simulink model "CuttingSim"  (R2021a)
settings: Solver=FixedStepAuto  StartTime=0.0  StopTime=Inf  RelTol=1e-3  EnableMultiTasking=on
model workspace (MAT data in the model file):
  SL_ROS_VariableLengthArrays_MaxSizes.CommonInfo.ArrayTruncateAction = 'EmitWarning'
  SL_ROS_VariableLengthArrays_MaxSizes.MsgTypeMap = containers.Map
  SL_ROS_VariableLengthArrays_MaxSizes.MsgTypeMap.serialization.keys = {'std_msgs/Float64MultiArray'}
  SL_ROS_VariableLengthArrays_MaxSizes.MsgTypeMap.serialization.values{1}.PropertyName = 'Data'
  SL_ROS_VariableLengthArrays_MaxSizes.MsgTypeMap.serialization.values{1}.DataType = 'double'
  SL_ROS_VariableLengthArrays_MaxSizes.MsgTypeMap.serialization.values{1}.MaxLength = 7
  SL_ROS_VariableLengthArrays_MaxSizes.MsgTypeMap.serialization.uniformity = 0
  SL_ROS_VariableLengthArrays_MaxSizes.MsgTypeMap.serialization.keyType = 'char'
  SL_ROS_VariableLengthArrays_MaxSizes.MsgTypeMap.serialization.valueType = 'any'
  q0 = Simulink.Parameter
  q0.Value = [-0.8706; 0.1348; 0.656; -1.7221; -0.0873; 1.3219; -0.1965]
  q0.DataType = 'auto'
  q0.Dimensions = [7 1]
  v_limit = 0.05
values from neighbouring files (symbols this model uses):
  Tf = 10    [createAgent.m]
  Ts = 0.02    [createAgent.m]
undefined symbols (not defined in the file or in its folder): rl
libraries: simulink x26, robotlib x8, vrlib x1, dspinverses x1, rllib x1, dspmathops x1
settings Model: ExtModeTrigMode=oneshot  ExtModeArmWhenConnect=off  Creator=pic  LastModifiedBy=workcell
settings SolverCC: AlgebraicLoopSolver=TrustRegion
settings DataIOCC: SaveFormat=StructureWithTime  SignalLoggingSaveFormat=ModelDataLogs
settings OptimizationCC: BlockReduction=off  BooleanDataType=off  EnhancedBackFolding=on  PassReuseOutputArgsThreshold=0  ExpressionDepthLimit=2147483647  InitFltsAndDblsToZero=on  MaxStackSize=64  OptimizeBlockOrder=speed  DifferentSizesBufferReuse=on  OptimizationCustomize=off
settings DebuggingCC: SaveWithParameterizedLinksMsg=none  UnderspecifiedInitializationDetection=Classic  MergeDetectMultiDrivingBlocksExec=none  SignalResolutionControl=TryResolveAllWithWarning  MultiTaskDSMMsg=warning  MultiTaskCondExecSysMsg=none  ParameterTunabilityLossMsg=error  FcnCallInpInsideContextMsg=warning  AllowSymbolicDim=off  StateNameClashWarn=warning  SFUnexpectedBacktrackingDiag=warning  SFNoUnconditionalDefaultTransitionDiag=warning  SFExecutionAtInitializationDiag=none  SFMachineParentedDataDiag=warning  ArithmeticOperatorsInVariantConditions=warning
settings HardwareCC: ProdBitPerPointer=32  ProdBitPerSizeT=32  ProdBitPerPtrDiffT=32  ProdLargestAtomicFloat=None  ProdIntDivRoundTo=Undefined  ProdEndianess=Unspecified  ProdWordSize=32  ProdHWDeviceType=Generic->Unspecified (assume 32-bit Generic)  TargetUnknown=on  UseEmbeddedCoderFeatures=off
settings ModelReferenceCC: PropagateSignalLabelsOutOfModel=off
settings SFSimCC: SimUseLocalCustomCode=off  MATLABDynamicMemAlloc=off  CustomCodeUndefinedFunction=UseInterfaceOnly  SimTargetLang=C++
settings RTWCC: SystemTargetFile=ert.tlc  HardwareBoard=Robot Operating System (ROS)  TLCOptions="-aInlineSetEventsForThisBaseRateFcn=TLC_FALSE -aSuppressMultiTaskScheduler=TLC_FALSE  -aRateBasedStepFcn=0"  TemplateMakefile=ert_default_tmf  RTWUseLocalCustomCode=off  Toolchain=Catkin  TargetLang=C++
settings CodeAppCC: ForceParamTrailComments=on  OperatorAnnotations=on
settings ERTTargetCC: ERTCustomFileBanners=off  SupportContinuousTime=on  SupportNonInlinedSFcns=on  RemoveResetFunc=off  ModelStepFunctionPrototypeControlCompliant=off
settings ConfigComp: CovMetricSettings=dw  CovSaveCumulativeToWorkspaceVar=on  CovSaveSingleToWorkspaceVar=on  CovExternalEMLEnable=off  CovSFcnEnable=off

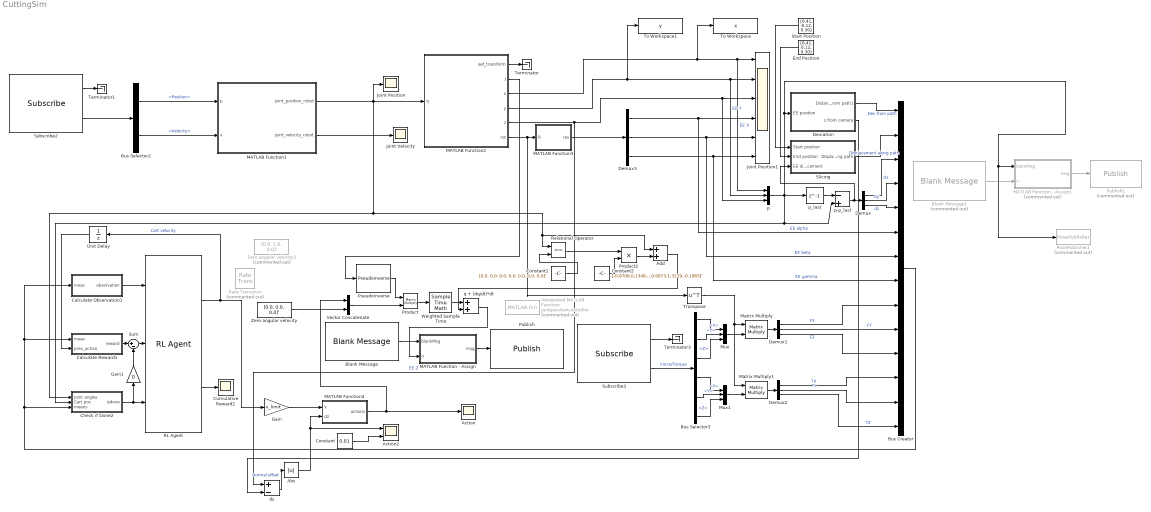
== system CuttingSim ==
  Abs : Abs
  Action : Scope
  Action2 : Scope  NumInputPorts=2
  Add : Sum
  Blank Message : robotlib/Blank Message  messageClass=Message  entityType=std_msgs/Float64MultiArray  messageType=std_msgs/Float64MultiArray  SampleTime=inf  legacyBusStruct=off
  Blank Message1 : robotlib/Blank Message  Commented=on  messageClass=Message  entityType=geometry_msgs/PoseStamped  messageType=geometry_msgs/PoseStamped  SampleTime=inf  legacyBusStruct=off
  Bus Creator : BusCreator  Inputs=14
  Bus Selector2 : BusSelector  OutputSignals=Position,Velocity
  Bus Selector3 : BusSelector  OutputSignals=Wrench.Force.X,Wrench.Force.Y,Wrench.Force.Z,Wrench.Torque.X,Wrench.Torque.Y,Wrench.Torque.Z
  Calculate Observation1 : Subsystem
  Calculate Reward1 : Subsystem
  Check if Done2 : Subsystem
  Constant : Constant  Value=0.01
  Constant1 : Constant  Value=[0.0, 0.0, 0.0, 0.0, 0.0, 0.0, 0.0]'
  Constant2 : Constant  Value=[-0.8706,0.1348,0.6560,-1.7221,-0.0873,1.3219,-0.1965]'
  Cumulative Reward2 : Scope
  Demux{,1..3} (4 alike) : Demux  Outputs=3
  Deviation : Subsystem
  End Position : Constant  Value=[0.41, 0.12, 0.30]  VectorParams1D=off
  Gain : Gain  Gain=v_limit
  Gain1 : Gain  Gain=0
  Interpreted MATLAB Function : MATLABFcn  Commented=on  MATLABFcn=jointpositioncontroller  OutputDimensions=0
  Joint Position : Scope
  Joint Position1 : Scope  NumInputPorts=6
  Joint Velocity : Scope
  MATLAB Function - Assign : MATLAB Function  TreatAsAtomicUnit=on
  MATLAB Function - Assign1 : MATLAB Function  Commented=on  TreatAsAtomicUnit=on
  MATLAB Function1 : MATLAB Function  TreatAsAtomicUnit=on
  MATLAB Function2 : MATLAB Function  TreatAsAtomicUnit=on
  MATLAB Function3 : MATLAB Function  TreatAsAtomicUnit=on
  MATLAB Function4 : MATLAB Function  TreatAsAtomicUnit=on
  Matrix Multiply : Product  Multiplication=Matrix(*)
  Matrix Multiply1 : Product  Multiplication=Matrix(*)
  Mux : Mux  Inputs=3
  Mux1 : Mux  Inputs=3
  PosePublisher1 : MATLABFcn  Commented=on  MATLABFcn=PosePublisher  OutputDimensions=0
  Product : Product  Multiplication=Matrix(*)
  Product2 : Product
  Pseudoinverse : dspinverses/Pseudoinverse  wanterr=off  SimulateUsing=Interpreted execution
      settings: SourceProductBaseCode=DS
  Publish : robotlib/Publish  topicSource=Select from ROS network  topic=/iiwa/PositionJointInterface_group_controller/command  messageType=std_msgs/Float64MultiArray  legacyBusStruct=off  messageQueueLength=1
  Publish1 : robotlib/Publish  Commented=on  topicSource=Select from ROS network  topic=/iiwa/PositionJointInterface_cutting_controller/CartesianPose  messageType=geometry_msgs/PoseStamped  legacyBusStruct=off  messageQueueLength=1
  RL Agent : rllib/RL Agent  Agent=rl.util.PolicyInstance.get('CuttingSim/RL Agent')  ExternalActionAsInput=off  ProvideCumRwd=on  TreatAsDirectFeedthrough=on
      settings: SourceProductName=Reinforcement Learning
  Rate Transition : RateTransition  Commented=on
  Relational Operator : RelationalOperator  Operator===  OutDataTypeStr=boolean  RndMeth=Simplest
  Slicing : Subsystem
  Start Position : Constant  Value=[0.41, -0.12, 0.30]  VectorParams1D=off
  Subscribe2 : robotlib/Subscribe  topicSource=Select from ROS network  topic=/iiwa/joint_states  messageType=sensor_msgs/JointState  SampleTime=-1  legacyBusStruct=off  messageQueueLength=1
  Subscribe3 : robotlib/Subscribe  topicSource=Select from ROS network  topic=/iiwa/CartesianWrench  messageType=geometry_msgs/WrenchStamped  SampleTime=-1  legacyBusStruct=off  messageQueueLength=1
  Sum : Sum  Inputs=|+-
  Terminator : Terminator
  Terminator1 : Terminator
  Terminator3 : Terminator
  To Workspace : ToWorkspace  VariableName=x  SaveFormat=Timeseries  SampleTime=-1
  To Workspace1 : ToWorkspace  VariableName=y  SaveFormat=Timeseries  SampleTime=-1
  Transpose : Math  Operator=transpose  SaturateOnIntegerOverflow=on
  Unit Delay : UnitDelay  SampleTime=-1  HasFrameUpgradeWarning=on
  Vector Concatenate : Concatenate
  Weighted Sample Time : SampleTimeMath  TsampMathOp=*
  Zero angular velocity : Constant  Value=[0.0, 0.0, 0.0]'
  Zero angular velocity1 : Constant  Commented=on  Value=[0.0, 1.0, 0.0]'
  dz : Sum  Inputs=+-
  p : Mux  Inputs=3
  p-p_last : Sum  Inputs=-+
  p_last : Delay  DelayLength=1  InitialCondition=0
  q + (dq/dt)*dt : Sum
  wires:
  Bus Creator/1 -> Check if Done2/3(means), Calculate Observation1/1(meas), Calculate Reward1/1(meas)
  Calculate Observation1/1(observation) -> RL Agent/1
  Check if Done2/1(isdone) -> RL Agent/3, Gain1/1
  RL Agent/1 -> Gain/1, Unit Delay/1  "Cart velocity"
  RL Agent/2 -> Cumulative Reward2/1
  Subscribe3/1 -> Terminator3/1
  Subscribe3/2 -> Bus Selector3/1  "Force/Torque"
  MATLAB Function2/3(x) -> To Workspace/1, Joint Position1/1, p/1  "EE X"
  MATLAB Function2/4(y) -> Joint Position1/2, p/2, To Workspace1/1  "EE Y"
  MATLAB Function2/5(z) -> p/3, Joint Position1/3, dz/1  "EE Z"
  Demux3/1 -> Bus Creator/6, Joint Position1/4  "EE alpha"
  Demux3/2 -> Bus Creator/7, Joint Position1/5  "EE beta"
  Demux3/3 -> Bus Creator/8, Joint Position1/6  "EE gamma"
  MATLAB Function2/6(rot) -> Transpose/1, MATLAB Function3/1(R)
  MATLAB Function3/1(res) -> Demux3/1
  Product/1 -> Weighted Sample Time/1
  Pseudoinverse/1 -> Product/1
  MATLAB Function2/2(J) -> Pseudoinverse/1
  Unit Delay/1 -> Calculate Reward1/2(prev_action)
  MATLAB Function2/1(eef_transform) -> Terminator/1
  p/1 -> PosePublisher1/1, MATLAB Function - Assign1/1(blankMsg), Deviation/1(EE position), Check if Done2/2(Cart pos), p-p_last/2, p_last/1
  End Position/1 -> Slicing/2(End position)
  Start Position/1 -> Slicing/1(Start position)
  Slicing/1(Displacement along path) -> Bus Creator/2  "Displacement along path"
  Deviation/1(Distance from path1) -> Bus Creator/1  "Dev from path"
  p_last/1 -> p-p_last/1
  p-p_last/1 -> Slicing/3(EE displacement), Demux/1
  Demux/1 -> Bus Creator/3  "dx"
  Demux/2 -> Bus Creator/4  "dy"
  Demux/3 -> Bus Creator/5  "dz"
  MATLAB Function1/1(joint_position_robot) -> Relational Operator/1, Add/1, Check if Done2/1(Joint angles), MATLAB Function2/1(q), Joint Position/1
  Subscribe2/2 -> Bus Selector2/1
  Bus Selector2/2 -> MATLAB Function1/2(v)  "<Velocity>"
  Bus Selector2/1 -> MATLAB Function1/1(p)  "<Position>"
  MATLAB Function1/2(joint_velocity_robot) -> Joint Velocity/1
  MATLAB Function - Assign/1(msg) -> Publish/1
  Blank Message/1 -> MATLAB Function - Assign/1(blankMsg)
  Subscribe2/1 -> Terminator1/1
  Bus Selector3/4 -> Mux1/1  "<X>"
  Bus Selector3/5 -> Mux1/2  "<Y>"
  Bus Selector3/6 -> Mux1/3  "<Z>"
  Bus Selector3/1 -> Mux/1  "<X>"
  Bus Selector3/2 -> Mux/2  "<Y>"
  Bus Selector3/3 -> Mux/3  "<Z>"
  Mux1/1 -> Matrix Multiply1/2
  Mux/1 -> Matrix Multiply/2
  Matrix Multiply1/1 -> Demux2/1
  Matrix Multiply/1 -> Demux1/1
  Demux1/1 -> Bus Creator/9  "FX"
  Demux1/2 -> Bus Creator/10  "FY"
  Demux1/3 -> Bus Creator/11  "FZ"
  Demux2/1 -> Bus Creator/12  "TX"
  Demux2/3 -> Bus Creator/14  "TZ"
  Demux2/2 -> Bus Creator/13  "TY"
  Transpose/1 -> Matrix Multiply1/1, Matrix Multiply/1
  Constant1/1 -> Relational Operator/2
  Relational Operator/1 -> Product2/1
  Product2/1 -> Add/2
  Constant2/1 -> Product2/2
  Add/1 -> q + (dq/dt)*dt/2
  Calculate Reward1/1(reward) -> Sum/1
  Sum/1 -> RL Agent/2
  Gain1/1 -> Sum/2
  Zero angular velocity/1 -> Vector Concatenate/2
  Vector Concatenate/1 -> Product/2
  Weighted Sample Time/1 -> q + (dq/dt)*dt/1
  q + (dq/dt)*dt/1 -> MATLAB Function - Assign/2(u)
  MATLAB Function - Assign1/1(msg) -> Publish1/1
  Blank Message1/1 -> MATLAB Function - Assign1/2(u)
  Deviation/2(z from camera) -> dz/2
  MATLAB Function4/1(actions) -> Vector Concatenate/1, Action/1
  Gain/1 -> MATLAB Function4/1(v)
  Abs/1 -> Action2/1, MATLAB Function4/2(dz)
  dz/1 -> Abs/1  "Normal offset"
  Constant/1 -> Action2/2

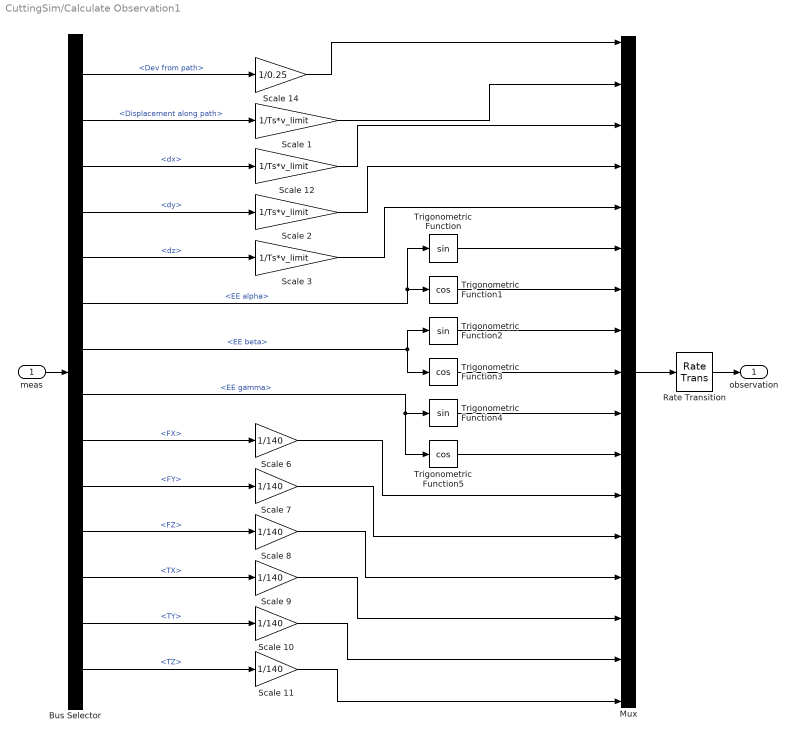
== system CuttingSim/Calculate Observation1 ==
  meas : Inport
  Bus Selector : BusSelector  OutputSignals=Dev from path,Displacement along path,dx,dy,dz,EE alpha,EE beta,EE gamma,FX,FY,FZ,TX,TY,TZ
  Mux : Mux  Inputs=17
  Rate Transition : RateTransition
  Scale {1..3,12} (4 alike) : Gain  Gain=1/Ts*v_limit
  Scale {6..11} (6 alike) : Gain  Gain=1/140
  Scale 14 : Gain  Gain=1/0.25
  Trigonometric Function : Trigonometry
  Trigonometric Function1 : Trigonometry  Operator=cos
  Trigonometric Function2 : Trigonometry
  Trigonometric Function3 : Trigonometry  Operator=cos
  Trigonometric Function4 : Trigonometry
  Trigonometric Function5 : Trigonometry  Operator=cos
  observation : Outport  VectorParamsAs1DForOutWhenUnconnected=off
  wires:
  meas/1 -> Bus Selector/1
  Mux/1 -> Rate Transition/1
  Bus Selector/1 -> Scale 14/1  "<Dev from path>"
  Scale 14/1 -> Mux/1
  Bus Selector/2 -> Scale 1/1  "<Displacement along path>"
  Scale 1/1 -> Mux/2
  Bus Selector/6 -> Trigonometric Function/1, Trigonometric Function1/1  "<EE alpha>"
  Bus Selector/7 -> Trigonometric Function2/1, Trigonometric Function3/1  "<EE beta>"
  Bus Selector/8 -> Trigonometric Function5/1, Trigonometric Function4/1  "<EE gamma>"
  Bus Selector/9 -> Scale 6/1  "<FX>"
  Trigonometric Function/1 -> Mux/6
  Trigonometric Function1/1 -> Mux/7
  Trigonometric Function2/1 -> Mux/8
  Trigonometric Function3/1 -> Mux/9
  Trigonometric Function5/1 -> Mux/11
  Trigonometric Function4/1 -> Mux/10
  Scale 6/1 -> Mux/12
  Rate Transition/1 -> observation/1
  Bus Selector/10 -> Scale 7/1  "<FY>"
  Scale 7/1 -> Mux/13
  Bus Selector/11 -> Scale 8/1  "<FZ>"
  Bus Selector/12 -> Scale 9/1  "<TX>"
  Bus Selector/13 -> Scale 10/1  "<TY>"
  Bus Selector/14 -> Scale 11/1  "<TZ>"
  Scale 8/1 -> Mux/14
  Scale 9/1 -> Mux/15
  Scale 10/1 -> Mux/16
  Scale 11/1 -> Mux/17
  Scale 12/1 -> Mux/3
  Bus Selector/3 -> Scale 12/1  "<dx>"
  Bus Selector/4 -> Scale 2/1  "<dy>"
  Bus Selector/5 -> Scale 3/1  "<dz>"
  Scale 2/1 -> Mux/4
  Scale 3/1 -> Mux/5

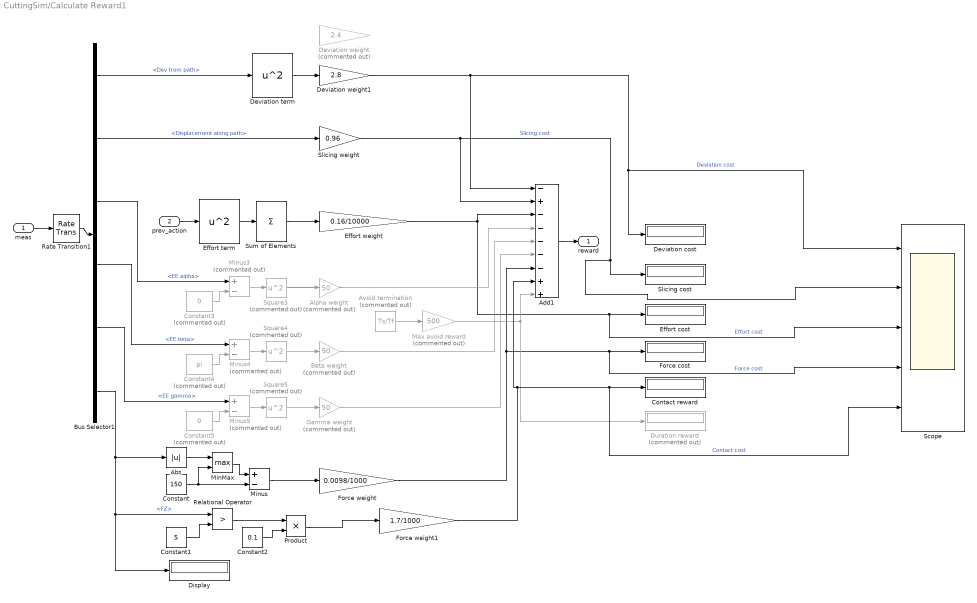
== system CuttingSim/Calculate Reward1 ==
  meas : Inport
  prev_action : Inport  Port=2
  Abs : Abs
  Add1 : Sum  Inputs=-+-----++
  Alpha weight : Gain  Commented=on  Gain=50
  Avoid termination : Constant  Commented=on  Value=Ts/Tf
  Beta weight : Gain  Commented=on  Gain=50
  Bus Selector1 : BusSelector  OutputSignals=Dev from path,Displacement along path,EE alpha,EE beta,EE gamma,FZ
  Constant : Constant  Value=150
  Constant1 : Constant  Value=5
  Constant2 : Constant  Value=0.1
  Constant3 : Constant  Commented=on  Value=0
  Constant4 : Constant  Commented=on  Value=pi
  Constant5 : Constant  Commented=on  Value=0
  Contact reward : Display
  Deviation cost : Display
  Deviation term : Math  Operator=square  SaturateOnIntegerOverflow=on
  Deviation weight : Gain  Commented=on  Gain=2.4
  Deviation weight1 : Gain  Gain=2.8
  Display : Display
  Duration reward : Display  Commented=on
  Effort cost : Display
  Effort term : Math  Operator=square  SaturateOnIntegerOverflow=on
  Effort weight : Gain  Gain=0.16/10000
  Force cost : Display
  Force weight : Gain  Gain=0.0098/1000
  Force weight1 : Gain  Gain=1.7/1000
  Gamma weight : Gain  Commented=on  Gain=50
  Max avoid reward : Gain  Commented=on  Gain=500
  MinMax : MinMax  Function=max  Inputs=2
  Minus : Sum  Inputs=+-
  Minus3 : Sum  Commented=on  Inputs=+-
  Minus4 : Sum  Commented=on  Inputs=+-
  Minus5 : Sum  Commented=on  Inputs=+-
  Product : Product
  Rate Transition1 : RateTransition  OutPortSampleTime=Ts
  Relational Operator : RelationalOperator  Operator=>  OutDataTypeStr=boolean  RndMeth=Simplest
  Scope : Scope  NumInputPorts=5
  Slicing cost : Display
  Slicing weight : Gain  Gain=0.96
  Square3 : Math  Commented=on  Operator=square  SignedPower=on  SaturateOnIntegerOverflow=on
  Square4 : Math  Commented=on  Operator=square  SignedPower=on  SaturateOnIntegerOverflow=on
  Square5 : Math  Commented=on  Operator=square  SignedPower=on  SaturateOnIntegerOverflow=on
  Sum of Elements : Sum  Inputs=+
  reward : Outport  VectorParamsAs1DForOutWhenUnconnected=off
  wires:
  meas/1 -> Rate Transition1/1
  Rate Transition1/1 -> Bus Selector1/1
  Add1/1 -> reward/1
  Minus3/1 -> Square3/1
  Constant3/1 -> Minus3/2
  Bus Selector1/3 -> Minus3/1  "<EE alpha>"
  Bus Selector1/4 -> Minus4/1  "<EE beta>"
  Constant4/1 -> Minus4/2
  Minus4/1 -> Square4/1
  Minus5/1 -> Square5/1
  Constant5/1 -> Minus5/2
  Bus Selector1/5 -> Minus5/1  "<EE gamma>"
  Sum of Elements/1 -> Effort weight/1
  Square3/1 -> Alpha weight/1
  Square4/1 -> Beta weight/1
  Square5/1 -> Gamma weight/1
  prev_action/1 -> Effort term/1
  Effort weight/1 -> Scope/3, Effort cost/1, Add1/3  "Effort cost"
  Deviation weight1/1 -> Add1/1, Scope/1, Deviation cost/1  "Deviation cost"
  Deviation term/1 -> Deviation weight1/1
  Bus Selector1/2 -> Slicing weight/1  "<Displacement along path>"
  Bus Selector1/1 -> Deviation term/1  "<Dev from path>"
  Effort term/1 -> Sum of Elements/1
  Bus Selector1/6 -> Relational Operator/1, Display/1, Abs/1  "<FZ>"
  Constant/1 -> Minus/2, MinMax/2
  Abs/1 -> MinMax/1
  MinMax/1 -> Minus/1
  Minus/1 -> Force weight/1
  Force weight/1 -> Add1/7, Scope/4, Force cost/1  "Force cost"
  Constant1/1 -> Relational Operator/2
  Relational Operator/1 -> Product/1
  Constant2/1 -> Product/2
  Product/1 -> Force weight1/1
  Alpha weight/1 -> Add1/4
  Beta weight/1 -> Add1/5
  Gamma weight/1 -> Add1/6
  Avoid termination/1 -> Max avoid reward/1
  Max avoid reward/1 -> Duration reward/1, Add1/9
  Force weight1/1 -> Add1/8, Scope/5, Contact reward/1  "Contact cost"
  Slicing weight/1 -> Add1/2, Scope/2, Slicing cost/1  "Slicing cost"

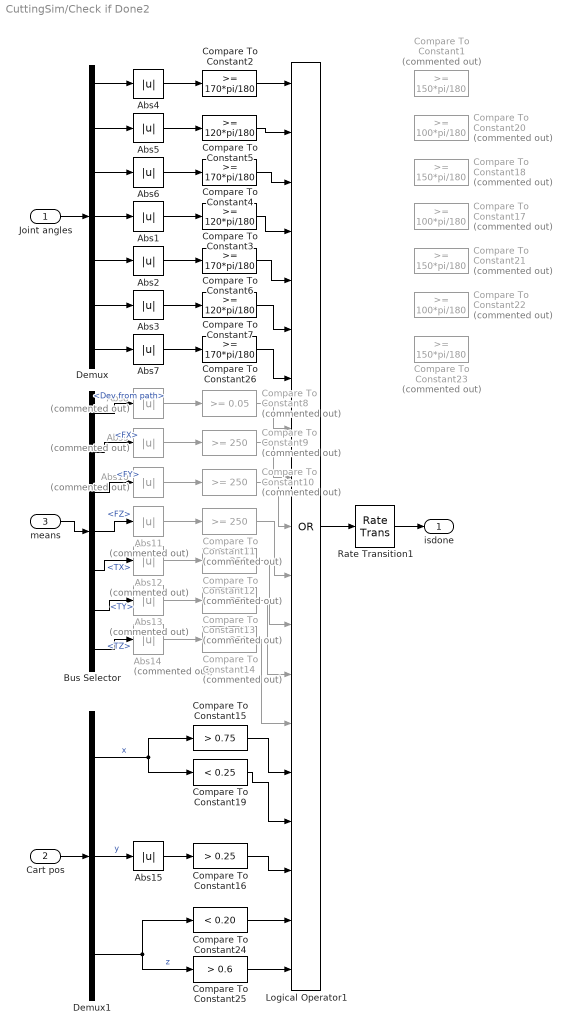
== system CuttingSim/Check if Done2 ==
  Joint angles : Inport
  Cart pos : Inport  Port=2
  means : Inport  Port=3
  Abs{1..7,15} (8 alike) : Abs
  Abs{8..14} (7 alike) : Abs  Commented=on
  Bus Selector : BusSelector  OutputSignals=Dev from path,FX,FY,FZ,TX,TY,TZ
  Compare To Constant{1,18,21,23} (4 alike) : simulink/Logic and Bit Operations/Compare To Constant  Commented=on  relop=>=  const=150*pi/180  OutDataTypeStr=boolean
  Compare To Constant{9..14} (6 alike) : simulink/Logic and Bit Operations/Compare To Constant  Commented=on  relop=>=  const=250  OutDataTypeStr=boolean
  Compare To Constant15 : simulink/Logic and Bit Operations/Compare To Constant  relop=>  const=0.75  OutDataTypeStr=boolean
  Compare To Constant16 : simulink/Logic and Bit Operations/Compare To Constant  relop=>  const=0.25  OutDataTypeStr=boolean
  Compare To Constant17 : simulink/Logic and Bit Operations/Compare To Constant  Commented=on  relop=>=  const=100*pi/180  OutDataTypeStr=boolean
  Compare To Constant19 : simulink/Logic and Bit Operations/Compare To Constant  relop=<  const=0.25  OutDataTypeStr=boolean
  Compare To Constant{2,4,6,26} (4 alike) : simulink/Logic and Bit Operations/Compare To Constant  relop=>=  const=170*pi/180  OutDataTypeStr=boolean
  Compare To Constant20 : simulink/Logic and Bit Operations/Compare To Constant  Commented=on  relop=>=  const=100*pi/180  OutDataTypeStr=boolean
  Compare To Constant22 : simulink/Logic and Bit Operations/Compare To Constant  Commented=on  relop=>=  const=100*pi/180  OutDataTypeStr=boolean
  Compare To Constant24 : simulink/Logic and Bit Operations/Compare To Constant  relop=<  const=0.20  OutDataTypeStr=boolean
  Compare To Constant25 : simulink/Logic and Bit Operations/Compare To Constant  relop=>  const=0.6  OutDataTypeStr=boolean
  Compare To Constant3 : simulink/Logic and Bit Operations/Compare To Constant  relop=>=  const=120*pi/180  OutDataTypeStr=boolean
  Compare To Constant5 : simulink/Logic and Bit Operations/Compare To Constant  relop=>=  const=120*pi/180  OutDataTypeStr=boolean
  Compare To Constant7 : simulink/Logic and Bit Operations/Compare To Constant  relop=>=  const=120*pi/180  OutDataTypeStr=boolean
  Compare To Constant8 : simulink/Logic and Bit Operations/Compare To Constant  Commented=on  relop=>=  const=0.05  OutDataTypeStr=boolean
  Demux : Demux  Outputs=7
  Demux1 : Demux  Outputs=3
  Logical Operator1 : Logic  Operator=OR  Inputs=19  AllPortsSameDT=off  OutDataTypeStr=boolean
  Rate Transition1 : RateTransition
  isdone : Outport  VectorParamsAs1DForOutWhenUnconnected=off
  wires:
  Compare To Constant8/1 -> Logical Operator1/8
  Demux/7 -> Abs7/1
  Compare To Constant26/1 -> Logical Operator1/7
  Demux/3 -> Abs6/1
  Demux/2 -> Abs5/1
  Abs3/1 -> Compare To Constant7/1
  Abs7/1 -> Compare To Constant26/1
  Compare To Constant3/1 -> Logical Operator1/4
  means/1 -> Bus Selector/1
  Abs8/1 -> Compare To Constant8/1
  Abs4/1 -> Compare To Constant2/1
  Demux/1 -> Abs4/1
  Rate Transition1/1 -> isdone/1
  Compare To Constant7/1 -> Logical Operator1/6
  Compare To Constant2/1 -> Logical Operator1/1
  Demux/5 -> Abs2/1
  Demux/6 -> Abs3/1
  Abs6/1 -> Compare To Constant4/1
  Abs2/1 -> Compare To Constant6/1
  Logical Operator1/1 -> Rate Transition1/1
  Compare To Constant5/1 -> Logical Operator1/2
  Abs1/1 -> Compare To Constant3/1
  Abs5/1 -> Compare To Constant5/1
  Compare To Constant6/1 -> Logical Operator1/5
  Joint angles/1 -> Demux/1
  Bus Selector/2 -> Abs9/1  "<FX>"
  Bus Selector/3 -> Abs10/1  "<FY>"
  Bus Selector/4 -> Abs11/1  "<FZ>"
  Bus Selector/5 -> Abs12/1  "<TX>"
  Bus Selector/7 -> Abs14/1  "<TZ>"
  Abs9/1 -> Compare To Constant9/1
  Abs10/1 -> Compare To Constant10/1
  Abs11/1 -> Compare To Constant11/1
  Abs12/1 -> Compare To Constant12/1
  Abs13/1 -> Compare To Constant13/1
  Bus Selector/6 -> Abs13/1  "<TY>"
  Abs14/1 -> Compare To Constant14/1
  Demux/4 -> Abs1/1
  Compare To Constant11/1 -> Logical Operator1/11
  Compare To Constant4/1 -> Logical Operator1/3
  Compare To Constant12/1 -> Logical Operator1/12
  Compare To Constant13/1 -> Logical Operator1/13
  Compare To Constant14/1 -> Logical Operator1/14
  Compare To Constant10/1 -> Logical Operator1/10
  Compare To Constant9/1 -> Logical Operator1/9
  Demux1/1 -> Compare To Constant19/1, Compare To Constant15/1  "x"
  Abs15/1 -> Compare To Constant16/1
  Demux1/2 -> Abs15/1  "y"
  Compare To Constant16/1 -> Logical Operator1/17
  Compare To Constant19/1 -> Logical Operator1/16
  Compare To Constant15/1 -> Logical Operator1/15
  Compare To Constant25/1 -> Logical Operator1/19
  Compare To Constant24/1 -> Logical Operator1/18
  Demux1/3 -> Compare To Constant25/1, Compare To Constant24/1  "z"
  Cart pos/1 -> Demux1/1
  Bus Selector/1 -> Abs8/1  "<Dev from path>"

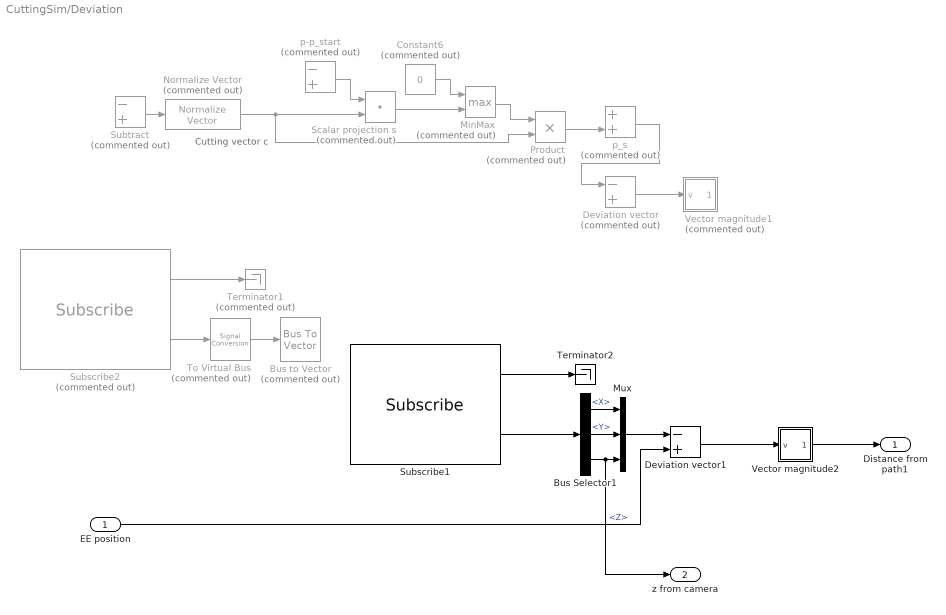
== system CuttingSim/Deviation ==
  note: Cutting vector c
  EE position : Inport
  Bus Selector1 : BusSelector  OutputSignals=Pose.Position.X,Pose.Position.Y,Pose.Position.Z
  Bus to Vector : BusToVector  Commented=on
  Constant6 : Constant  Commented=on  Value=0
  Deviation vector : Sum  Commented=on  Inputs=-+
  Deviation vector1 : Sum  Inputs=-+
  MinMax : MinMax  Commented=on  Function=max  Inputs=2  OutMin=[0]
  Mux : Mux  Inputs=3
  Normalize Vector : vrlib/Utilities/Normalize Vector  Commented=on  maxzero=0
  Product : Product  Commented=on
  Scalar projection s : DotProduct  Commented=on  InputSameDT=on  OutDataTypeStr=Inherit: Inherit via internal rule
  Subscribe1 : robotlib/Subscribe  topicSource=Select from ROS network  topic=/iiwa/CartesianPose/surface  messageType=geometry_msgs/PoseStamped  SampleTime=-1  legacyBusStruct=off  messageQueueLength=1
  Subscribe2 : robotlib/Subscribe  Commented=on  topicSource=Select from ROS network  topic=/iiwa/CartesianPose/surface  messageType=geometry_msgs/PoseStamped  SampleTime=-1  legacyBusStruct=off  messageQueueLength=1
  Subtract : Sum  Commented=on  Inputs=-+
  Terminator1 : Terminator  Commented=on
  Terminator2 : Terminator
  To Virtual Bus : SignalConversion  Commented=on  ConversionOutput=Virtual bus  OverrideOpt=off
  Vector magnitude1 : Subsystem  Commented=on
  Vector magnitude2 : Subsystem
  p-p_start : Sum  Commented=on  Inputs=-+
  p_s : Sum  Commented=on
  Distance from path1 : Outport
  z from camera : Outport  Port=2
  wires:
  Product/1 -> p_s/2
  Subtract/1 -> Normalize Vector/1
  p-p_start/1 -> Scalar projection s/1
  Scalar projection s/1 -> MinMax/2
  Constant6/1 -> MinMax/1
  MinMax/1 -> Product/1
  p_s/1 -> Deviation vector/1
  Normalize Vector/1 -> Product/2, Scalar projection s/2
  Deviation vector/1 -> Vector magnitude1/1(v)
  EE position/1 -> Deviation vector1/2
  Vector magnitude2/1(||v||) -> Distance from path1/1
  Subscribe2/1 -> Terminator1/1
  To Virtual Bus/1 -> Bus to Vector/1
  Subscribe2/2 -> To Virtual Bus/1
  Mux/1 -> Deviation vector1/1
  Subscribe1/1 -> Terminator2/1
  Bus Selector1/1 -> Mux/1  "<X>"
  Subscribe1/2 -> Bus Selector1/1
  Bus Selector1/2 -> Mux/2  "<Y>"
  Deviation vector1/1 -> Vector magnitude2/1(v)
  Bus Selector1/3 -> z from camera/1, Mux/3  "<Z>"

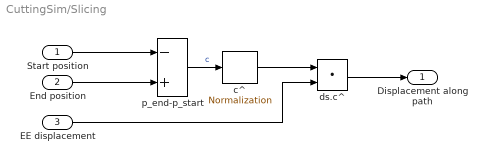
== system CuttingSim/Slicing ==
  Start position : Inport
  End position : Inport  Port=2
  EE displacement : Inport  Port=3
  c^ : dspmathops/Normalization  NormType=2-norm  Bias=1e-10  NormOver=Each column  Dimension=1  roundingMode=Floor  overflowMode=off  accumDataTypeStr=Inherit: Same as product output  accumLastDataTypeStr=Inherit: Same as product output  outputDataTypeStr=Inherit: Same as product output  outputMin=[]  outputMax=[]  outputLastDataTypeStr=Inherit: Same as product output
  ds.c^ : DotProduct  InputSameDT=on  OutDataTypeStr=Inherit: Inherit via internal rule
  p_end-p_start : Sum  Inputs=-+
  Displacement along path : Outport
  wires:
  Start position/1 -> p_end-p_start/1
  End position/1 -> p_end-p_start/2
  p_end-p_start/1 -> c^/1  "c"
  EE displacement/1 -> ds.c^/2
  c^/1 -> ds.c^/1
  ds.c^/1 -> Displacement along path/1

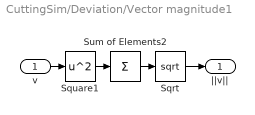
== system CuttingSim/Deviation/Vector magnitude1 ==
  v : Inport
  Sqrt : Sqrt  SaturateOnIntegerOverflow=on
  Square1 : Math  Operator=square  SaturateOnIntegerOverflow=on
  Sum of Elements2 : Sum  Inputs=+
  ||v|| : Outport
  wires:
  Sqrt/1 -> ||v||/1
  Sum of Elements2/1 -> Sqrt/1
  Square1/1 -> Sum of Elements2/1
  v/1 -> Square1/1

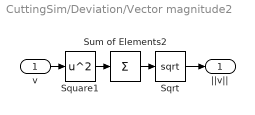
== system CuttingSim/Deviation/Vector magnitude2 ==
  v : Inport
  Sqrt : Sqrt  SaturateOnIntegerOverflow=on
  Square1 : Math  Operator=square  SaturateOnIntegerOverflow=on
  Sum of Elements2 : Sum  Inputs=+
  ||v|| : Outport
  wires:
  Sqrt/1 -> ||v||/1
  Sum of Elements2/1 -> Sqrt/1
  Square1/1 -> Sum of Elements2/1
  v/1 -> Square1/1

== matlab function CuttingSim/MATLAB Function2 ==
  data: q input; eef_transform output; J output; x output; y output; z output; rot output
%function [eef_transform,J,x,y,z,rot]=directKinematics(q1,q2,q3,q4,q5,q6,q7)
function [eef_transform,J,x,y,z,rot]=directKinematics(q)
% DH PARAMETERS FOR THE ROBOT
alfa={0,-pi/2,pi/2,pi/2,-pi/2,-pi/2,pi/2};
%q=[q1,q2,q3,q4,q5,q6,q7];
d={0.36,0.0,0.42,0.0,0.4,0.0,0.126};
d{7}=0.020+0.34017; 
a={0,0,0,0,0,0,0};

%% Calculating the direct Kinematics
T=zeros(4,4,7);
i=1;
T(:,:,i)=getDHMatrix(alfa{i},q(i),d{i},a{i});
    for i=2:7
        T(:,:,i)=T(:,:,i-1)*getDHMatrix(alfa{i},q(i),d{i},a{i});
        T(:,:,i)=normalizeColumns(T(:,:,i));
    end
        T(:,:,7)=T(:,:,7);
        T(:,:,7)=normalizeColumns(T(:,:,7));
        
    pef=T(1:3,4,7);
    J=zeros(6,7);
    for i=1:7
        k=T(1:3,3,i);
        pij=pef-T(1:3,4,i);
        J(1:3,i)=cross(k,pij);
        J(4:6,i)=k;
    end
%% End effector transform
eef_transform=T(:,:,7);
x=T(1,4,7);
y=T(2,4,7);
z=T(3,4,7);
rot=T(1:3,1:3,7);
end

function T=getDHMatrix(alfa,theta,d,a)
T=zeros(4,4);
calpha=cos(alfa);
sinalpha=sin(alfa);
coshteta=cos(theta);
sintheta=sin(theta);

T(1,1)=coshteta;
T(2,1)=sintheta*calpha;
T(3,1)=sintheta*sinalpha;				

T(1,2)=-sintheta;
T(2,2)=coshteta*calpha;
T(3,2)=coshteta*sinalpha;

T(2,3)=-sinalpha;
T(3,3)=calpha;

T(1,4)=a;
T(2,4)=-sinalpha*d;
T(3,4)=calpha*d;
T(4,4)=1;

end

function normalizedT=normalizeColumns(T)

r=zeros(4,3); % corrected rotatio matrix, with zero badding row at the end
for j=1:3
    r(1:3,j)=T(1:3,j)/norm(T(1:3,j));
end
normalizedT=[r,T(:,4)];
end

== matlab function CuttingSim/MATLAB Function - Assign ==
  data: blankMsg input; u input; msg output Bus: SL_Bus_CuttingSim_std_msgs_Float64MultiArray
function msg = assign(blankMsg, u)
% Copyright 2021 The MathWorks, Inc.
%#codegen

% To set datatype of MSG output:
%  1. Create buses for this model: robotics.ros.createSimulinkBus(gcs)
%  1. Click "Edit Data" in  Toolstrip to open "Ports and Data Manager"
%  2. Select MSG and set datatype to "Bus: SL_Bus_<modelname>_<messageType>"
% See: 
% http://www.mathworks.com/help/simulink/ug/create-structures-in-matlab-function-blocks.html

% Assign the output message to be the same with input blank message
msg = blankMsg;

% Modify the nested Pose and Twist messages
msg.Data(1:numel(u)) = reshape(u,[],1);
msg.Data_SL_Info.CurrentLength = uint32(numel(u));
msg.Layout.Dim(1).Size = uint32(size(u,1));
msg.Layout.Dim(2).Size = uint32(size(u,2));
msg.Layout.Dim(1).Stride = uint32(prod(size(u)));
msg.Layout.Dim(2).Stride = uint32(prod(size(u,2)));

== matlab function CuttingSim/MATLAB Function - Assign1 ==
  data: blankMsg input; u input; msg output Bus: SL_Bus_CuttingSim_std_msgs_Float64MultiArray
function msg = assign(blankMsg, u)
% Copyright 2021 The MathWorks, Inc.
%#codegen

% To set datatype of MSG output:
%  1. Create buses for this model: robotics.ros.createSimulinkBus(gcs)
%  1. Click "Edit Data" in  Toolstrip to open "Ports and Data Manager"
%  2. Select MSG and set datatype to "Bus: SL_Bus_<modelname>_<messageType>"
% See: 
% http://www.mathworks.com/help/simulink/ug/create-structures-in-matlab-function-blocks.html

% Assign the output message to be the same with input blank message
msg = blankMsg;

% Modify the nested Pose and Twist messages
msg.Data(1:numel(u)) = reshape(u,[],1);
msg.Data_SL_Info.CurrentLength = uint32(numel(u));
msg.Layout.Dim(1).Size = uint32(size(u,1));
msg.Layout.Dim(2).Size = uint32(size(u,2));
msg.Layout.Dim(1).Stride = uint32(prod(size(u)));
msg.Layout.Dim(2).Stride = uint32(prod(size(u,2)));

== matlab function CuttingSim/MATLAB Function3 ==
  data: R input; res output
function res=rot2eulZYX(R)
    [res]=eulerAngles(R) ;
end

function y=closeEnough(a,b)
    epsilon=0.000001;
    if (epsilon>abs(a-b))
        y=1;
    else
        y=0;
    end
end

function [res]=eulerAngles(R) 
    %% check for gimbal lock
    R=R';
    if (closeEnough(R(1,3), -1.0)) 
        b = 0; %% gimbal lock, value of x doesn't matter
        c = pi / 2;
        a = b + atan2(R(2,1), R(3,1));
    elseif (closeEnough(R(1,3), 1.0)) 
        b = 0;
        c = -pi / 2;
        a = -b + atan2(-R(2,1), -R(3,1));
    else  %% two solutions exist
        b1 = -asin(R(1,3));
        b2 = pi - b1;

        c1 = atan2(R(2,3) / cos(b1), R(3,3) / cos(b1));
        c2 = atan2(R(2,3) / cos(b2), R(3,3) / cos(b2));

        a1 = atan2(R(1,2) / cos(b1), R(1,1)/ cos(b1));
        a2 = atan2(R(1,2) / cos(b2), R(1,1) / cos(b2));

        %% choose one solution to return
        %% for example the "shortest" rotation
        condition=((abs(b1) + abs(c1) + abs(a1)) <= (abs(b2) + abs(c2) + abs(a2)));
        if condition 
            a=a1;
            b=b1;
            c=c1;   
        else 
            a=a2;
            b=b2;
            c=c2;   
        end
    end
    res=[a,b,c];
end

== matlab function CuttingSim/MATLAB Function4 ==
  data: v input; actions output; dz input
function actions = vel(v,dz)


if dz < 0.005
    actions =  v ; 
 else
     actions = [v(1),v(2),0]' ;
 end
 
end

== matlab function CuttingSim/MATLAB Function1 ==
  data: joint_position_robot output; joint_velocity_robot output; p input; v input
function  [joint_position_robot,joint_velocity_robot]=states(p,v)
joint_position_robot=[p(1),p(2),p(3),p(4),p(5),p(6),p(7)]';
joint_velocity_robot=[v(1),v(2),v(3),v(4),v(5),v(6),v(7)]';         
end
